simulink model "Task3_2"  (R2018b)
settings: Solver=VariableStepAuto  StartTime=0.0  StopTime=15  RelTol=1e-3
settings Model: Creator=Федор  LastModifiedBy=Федор
settings SolverCC: ZeroCrossAlgorithm=Adaptive
settings DebuggingCC: IgnoredZcDiagnostic=none

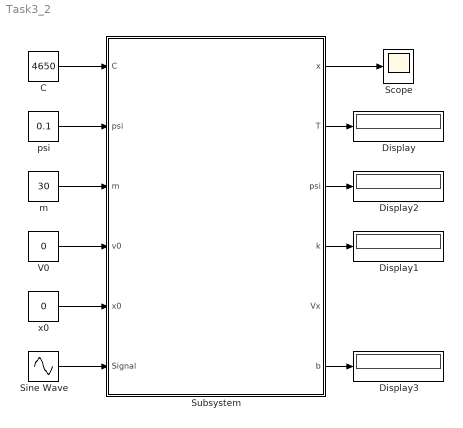
== system Task3_2 ==
  C : Constant  Value=4650
  Display{,1..3} (4 alike) : Display
  Scope : Scope
  Sine Wave : Sin  Amplitude=100  Frequency=12.45  SampleTime=0
  Subsystem : Subsystem
  "V0 " : Constant  Value=0
  "m " : Constant  Value=30
  psi : Constant  Value=0.1
  "x0 " : Constant  Value=0
  wires:
  C/1 -> Subsystem/1(C)
  psi/1 -> Subsystem/2("psi ")
  "m "/1 -> Subsystem/3(m)
  "V0 "/1 -> Subsystem/4(v0)
  "x0 "/1 -> Subsystem/5(x0)
  Sine Wave/1 -> Subsystem/6("Signal ")
  Subsystem/1(x) -> Scope/1
  Subsystem/2(T) -> Display/1
  Subsystem/3(psi) -> Display2/1
  Subsystem/4(k) -> Display1/1
  Subsystem/6(b) -> Display3/1

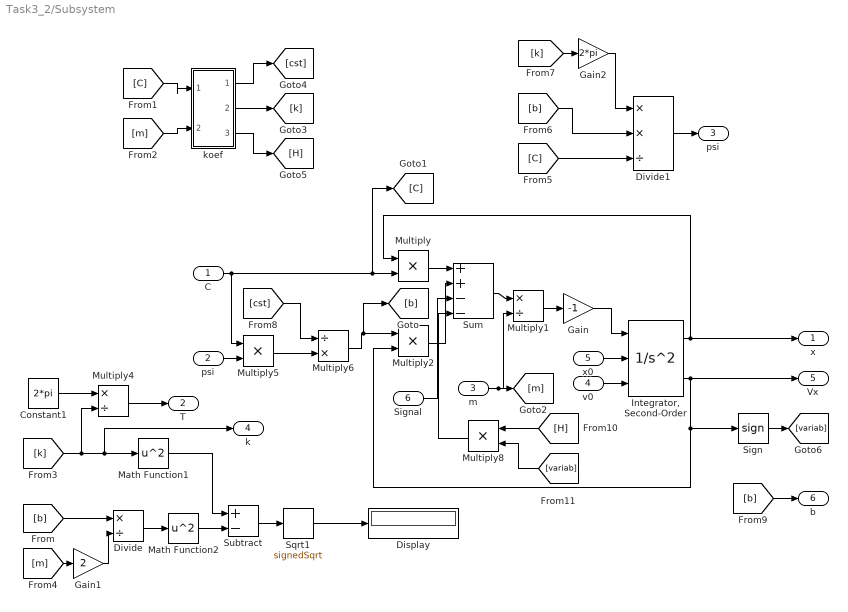
== system Task3_2/Subsystem ==
  C : Inport
  "psi " : Inport  Port=2
  m : Inport  Port=3
  v0 : Inport  Port=4
  x0 : Inport  Port=5
  "Signal " : Inport  Port=6
  Constant1 : Constant  Value=2*pi
  Display : Display
  Divide : Product  Inputs=*/  OutDataTypeStr=double
  Divide1 : Product  Inputs=**/  OutDataTypeStr=double
  Gain : Gain  Gain=-1
  Gain1 : Gain  Gain=2
  Gain2 : Gain  Gain=2*pi
  "Integrator, Second-Order" : SecondOrderIntegrator  ICSourceX=external  ICSourceDXDT=external
  Math Function1 : Math  Operator=square  OutDataTypeStr=double  SaturateOnIntegerOverflow=on
  Math Function2 : Math  Operator=square  SaturateOnIntegerOverflow=on
  Multiply{,2,5,8} (4 alike) : Product
  Multiply1 : Product  Inputs=*/
  Multiply4 : Product  Inputs=*/
  Multiply6 : Product  Inputs=/*
  Sign : Signum
  Sqrt1 : Sqrt  Operator=signedSqrt  SaturateOnIntegerOverflow=on
  Subtract : Sum  Inputs=+-  OutDataTypeStr=double
  Sum : Sum  Inputs=++--
  koef : Subsystem
  x : Outport
  T : Outport  Port=2
  psi : Outport  Port=3
  k : Outport  Port=4
  Vx : Outport  Port=5
  b : Outport  Port=6
  wires:
  Gain/1 -> "Integrator, Second-Order"/1
  "Integrator, Second-Order"/1 -> Multiply/1, x/1
  Multiply1/1 -> Gain/1
  m/1 -> Multiply1/2, [m]
  Multiply/1 -> Sum/1
  Multiply2/1 -> Sum/2
  Sum/1 -> Multiply1/1
  "Integrator, Second-Order"/2 -> Vx/1, Sign/1, Multiply2/2
  v0/1 -> "Integrator, Second-Order"/3
  "Signal "/1 -> Sum/3
  C/1 -> Multiply5/1, [C], Multiply/2
  x0/1 -> "Integrator, Second-Order"/2
  Constant1/1 -> Multiply4/1
  Multiply4/1 -> T/1
  [k] -> k/1, Math Function1/1, Multiply4/2
  [m] -> Gain1/1
  [b] -> Divide/1
  Gain1/1 -> Divide/2
  Divide/1 -> Math Function2/1
  Math Function2/1 -> Subtract/2
  Subtract/1 -> Sqrt1/1
  Sqrt1/1 -> Display/1
  Gain2/1 -> Divide1/1
  [C] -> Divide1/3
  [b] -> Divide1/2
  Divide1/1 -> psi/1
  Math Function1/1 -> Subtract/1
  [k] -> Gain2/1
  "psi "/1 -> Multiply5/2
  Multiply5/1 -> Multiply6/2
  [cst] -> Multiply6/1
  Multiply6/1 -> [b], Multiply2/1
  [b] -> b/1
  Multiply8/1 -> Sum/4
  Sign/1 -> [variab]
  [H] -> Multiply8/1
  [variab] -> Multiply8/2
  [C] -> koef/1(In1)
  [m] -> koef/2(In2)
  koef/1(Out1) -> [cst]
  koef/2(Out2) -> [k]
  koef/3(Out3) -> [H]

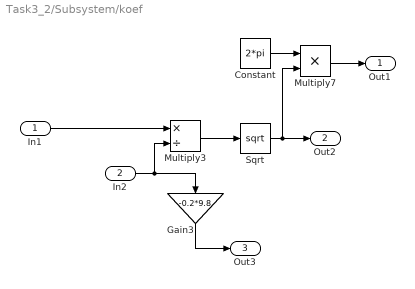
== system Task3_2/Subsystem/koef ==
  In1 : Inport
  In2 : Inport  Port=2
  Constant : Constant  Value=2*pi
  Gain3 : Gain  Gain=-0.2*9.8
  Multiply3 : Product  Inputs=*/
  Multiply7 : Product
  Sqrt : Sqrt  SaturateOnIntegerOverflow=on
  Out1 : Outport
  Out2 : Outport  Port=2
  Out3 : Outport  Port=3
  wires:
  In1/1 -> Multiply3/1
  Gain3/1 -> Out3/1
  In2/1 -> Gain3/1, Multiply3/2
  Constant/1 -> Multiply7/1
  Sqrt/1 -> Out2/1, Multiply7/2
  Multiply3/1 -> Sqrt/1
  Multiply7/1 -> Out1/1
